simulink model "Pollution"  (Simulink 10.0)
settings: Solver=ode45  StartTime=0.0  StopTime=10.0  RelTol=1e-3  EnableMultiTasking=on
settings Model: Creator=tjohnson  LastModifiedBy=unknown
settings DataIOCC: LimitDataPoints=on
settings DebuggingCC: UnderspecifiedInitializationDetection=Simplified  MergeDetectMultiDrivingBlocksExec=error
settings GRTTargetCC: GeneratePreprocessorConditionals=Disable all  CombineOutputUpdateFcns=on  GRTInterface=off
settings ConfigComp: CovExternalEMLEnable=off

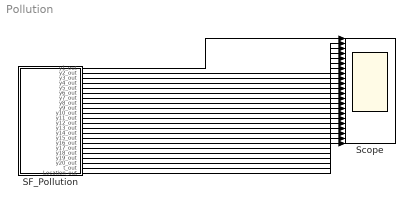
== system Pollution ==
  SF_Pollution : Stateflow chart  TreatAsAtomicUnit=on
  Scope : Scope  NumInputPorts=22
  wires:
  SF_Pollution/1(y1_out) -> Scope/1
  SF_Pollution/2(y2_out) -> Scope/2
  SF_Pollution/3(y3_out) -> Scope/3
  SF_Pollution/4(y4_out) -> Scope/4
  SF_Pollution/5(y5_out) -> Scope/5
  SF_Pollution/6(y6_out) -> Scope/6
  SF_Pollution/7(y7_out) -> Scope/7
  SF_Pollution/8(y8_out) -> Scope/8
  SF_Pollution/9(y9_out) -> Scope/9
  SF_Pollution/10(y10_out) -> Scope/10
  SF_Pollution/11(y11_out) -> Scope/11
  SF_Pollution/12(y12_out) -> Scope/12
  SF_Pollution/13(y13_out) -> Scope/13
  SF_Pollution/14(y14_out) -> Scope/14
  SF_Pollution/15(y15_out) -> Scope/15
  SF_Pollution/16(y16_out) -> Scope/16
  SF_Pollution/17(y17_out) -> Scope/17
  SF_Pollution/18(y18_out) -> Scope/18
  SF_Pollution/19(y19_out) -> Scope/19
  SF_Pollution/20(y20_out) -> Scope/20
  SF_Pollution/21(t_out) -> Scope/21
  SF_Pollution/22(Location_out) -> Scope/22

== stateflow chart SF_Pollution ==
  settings: updateMethod=CONTINUOUS
  state pollution
    du:
    y1_dot = -k1 * y1 - k10 * y11 * y1 - k14 * y1 * y6 - k23 * y1 * y4 - k24 * y19 * y1 + k2 * y2 * y4 + k3 * y5 * y2 + k9 * y11 * y2 + k11 * y13 + k12 * y10 * y2 + k22 * y19 + k25 * y20;
    y2_dot = -k2 * y2 * y4 - k3 * y5 * y2 - k9 * y11 * y2 - k12 * y10 * y2 + k1 * y1 + k21 * y19;
    y3_dot = -k15 * y3 + k1 * y1 + k17 * y4 + k19 * y16 + k22 * y19;
    y4_dot = -k2 * y2 * y4 - k16 * y4 - k17 * y4 - k23 * y1 * y4 + k15 * y3;
    y5_dot = -k3 * y5 * y2 + 2.0 * k4 * y7 + k6 * y7 * y6 + k7 * y9 + k13 * y14 + k20 * y17 * y6;
    y6_dot = -k6 * y7 * y6 - k8 * y9 * y6 - k14 * y1 * y6 - k20 * y17 * y6 + k3 * y5 * y2 + 2.0 * k18 * y16;
    y7_dot = -k4 * y7 - k5 * y7 - k6 * y7 * y6 + k13 * y14;
    y8_dot = k4 * y7 + k5 * y7 + k6 * y7 * y6 + k7 * y9;
    y9_dot = -k7 * y9 - k8 * y9 * y6;
    y10_dot = -k12 * y10 * y2 + k7 * y9 + k9 * y11 * y2;
    y11_dot = -k9 * y11 * y2 - k10 * y11 * y1 + k8 * y9 * y6 + k11 * y13;
    y12_dot = k9 * y11 * y2;
    y13_dot = -k11 * y13 + k10 * y11 * y1;
    y14_dot = -k13 * y14 + k12 * y10 * y2;
    y15_dot = k14 * y1 * y6;
    y16_dot = -k18 * y16 - k19 * y16 + k16 * y4;
    y17_dot = -k20 * y17 * y6;
    y18_dot = k20 * y17 * y6;
    y19_dot = -k21 * y19 - k22 * y19 - k24 * y19 * y1 + k23 * y1 * y4 + k25 * y20;
    y20_dot = -k25 * y20 + k24 * y19 * y1;
    t_dot = 1.0;
    y1_out=y1;
    y2_out=y2;
    y3_out=y3;
    y4_out=y4;
    y5_out=y5;
    y6_out=y6;
    y7_out=y7;
    y8_out=y8;
    y9_out=y9;
    y10_out=y10;
    y11_out=y11;
    y12_out=y12;
    y13_out=y13;
    y14_out=y14;
    y15_out=y15;
    y16_out=y16;
    y17_out=y17;
    y18_out=y18;
    y19_out=y19;
    y20_out=y20;
    t_out=t;
    Location_out =1;
  (default) -> pollution : {t = 0.0; y1 = 0.0; y10 = 0.0; y11 = 0.0; y12 = 0.0; y13 = 0.0; y14 = 0.0; y15 = 0.0; y16 = 0.0; y17 = 0.007; y18 = 0.0; y19 = 0.0; y2 = 0.2; y20 = 0.0; y3 = 0.0; y4 = 0.04; y5 = 0.0; y6 = 0.0; y7 = 0.1; y8 = 0.3; y9 = 0.01;}
  data: k1 constant double =0.35; k2 constant double =26.6; k3 constant double =12300; k4 constant double =0.00086; k5 constant double =0.00082; k6 constant double =15000; k7 constant double =0.00013; k8 constant double =24000; k9 constant double =16500; k10 constant double =9000; k11 constant double =0.022; k12 constant double =12000; k13 constant double =1.88; k14 constant double =16300; k15 constant double =4800000; k16 constant double =0.00035; k17 constant double =0.0175; k18 constant double =100000000; k19 constant double =444000000000; k20 constant double =1240; k21 constant double =2.1; k22 constant double =5.78; k23 constant double =0.0474; k24 constant double =1780; k25 constant double =3.12; stop_time constant double =15; y1 local double; y1_out output double; y2 local double; y2_out output double; y3 local double; y3_out output double; y4 local double; y4_out output double; y5 local double; y5_out output double; y6 local double; y6_out output double; y7 local double; y7_out output double; y8 local double; y8_out output double; y9 local double; y9_out output double; y10 local double; y10_out output double; y11 local double; y11_out output double; y12 local double; y12_out output double; y13 local double; y13_out output double; y14 local double; y14_out output double; y15 local double; y15_out output double; y16 local double; y16_out output double; y17 local double; y17_out output double; y18 local double; y18_out output double; y19 local double; y19_out output double; y20 local double; y20_out output double; t local double; t_out output double; Location_out output double
  data y1 settings: updateMethod=SF_CONTINUOUS_TIME_DATA
  data y2 settings: updateMethod=SF_CONTINUOUS_TIME_DATA
  data y3 settings: updateMethod=SF_CONTINUOUS_TIME_DATA
  data y4 settings: updateMethod=SF_CONTINUOUS_TIME_DATA
  data y5 settings: updateMethod=SF_CONTINUOUS_TIME_DATA
  data y6 settings: updateMethod=SF_CONTINUOUS_TIME_DATA
  data y7 settings: updateMethod=SF_CONTINUOUS_TIME_DATA
  data y8 settings: updateMethod=SF_CONTINUOUS_TIME_DATA
  data y9 settings: updateMethod=SF_CONTINUOUS_TIME_DATA
  data y10 settings: updateMethod=SF_CONTINUOUS_TIME_DATA
  data y11 settings: updateMethod=SF_CONTINUOUS_TIME_DATA
  data y12 settings: updateMethod=SF_CONTINUOUS_TIME_DATA
  data y13 settings: updateMethod=SF_CONTINUOUS_TIME_DATA
  data y14 settings: updateMethod=SF_CONTINUOUS_TIME_DATA
  data y15 settings: updateMethod=SF_CONTINUOUS_TIME_DATA
  data y16 settings: updateMethod=SF_CONTINUOUS_TIME_DATA
  data y17 settings: updateMethod=SF_CONTINUOUS_TIME_DATA
  data y18 settings: updateMethod=SF_CONTINUOUS_TIME_DATA
  data y19 settings: updateMethod=SF_CONTINUOUS_TIME_DATA
  data y20 settings: updateMethod=SF_CONTINUOUS_TIME_DATA
  data t settings: updateMethod=SF_CONTINUOUS_TIME_DATA
